simulink model "OpInvDyn"  (Simulink 7.4)
settings: Solver=ode45  StartTime=0.0  StopTime=8  MinStep=0.01  RelTol=1e-3
values from neighbouring files (symbols this model uses):
  Kd = Kp.^0.5*2    [WAMforcecontrol.m]    (also in batchwamobs.m = 50*eye(7); paralelcontrol2R.m = eye(n)*1000)
  Kp = 25*eye(7)    [batchwamobs.m]    (also in paralelcontrol2R.m = eye(n)*2500)
  Md = eye(n)*5    [WAMforcecontrol.m]    (also in feedforward.m = inertia(robot, qd(i,:)); paralelcontrol2R.m = eye(n)*100)
undefined symbols (not defined in the file or in its folder): fdbckOID, p560, splitsignal
libraries: roblocks x2
settings Model: Creator=acolome  LastModifiedBy=acolome

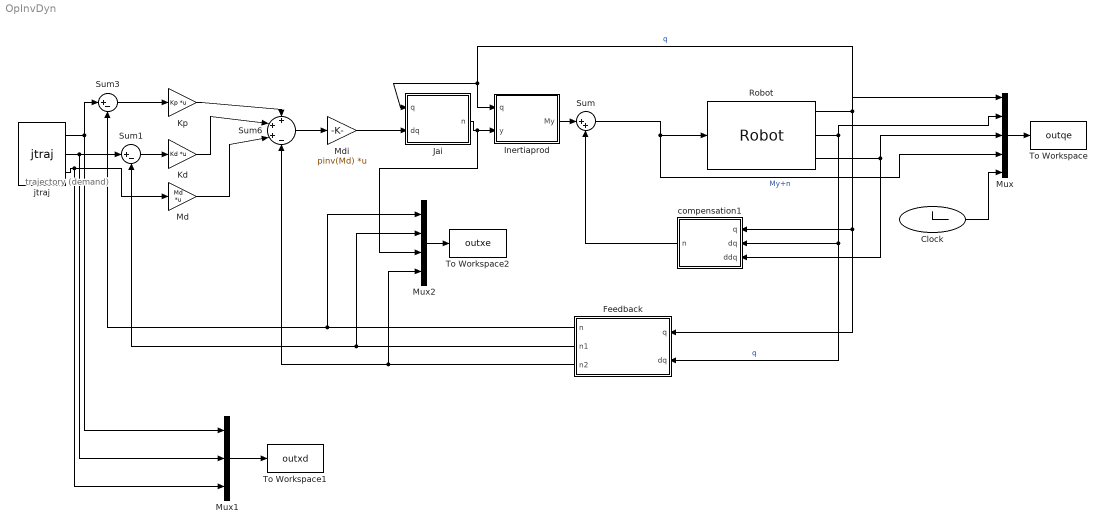
== system OpInvDyn ==
  note: trajectory
      | (demand)
  Clock : Clock
      settings: Decimation=100
  Feedback : Subsystem  mask{robot=p560, g=[0 0 9.81]}
      mask prompts: robot "Robot Object"; g "Gravity"
      mask init:
      | n=robot.n
      mask Display:
      | port_label('output',1,'xe')
      | port_label('output',2,'dxe')
      | port_label('output',3,'dJ(q,dq)·dq')
      | 
      | port_label('input', 1, 'q')
      | port_label('input', 2, 'dq')
  Inertiaprod : Subsystem  mask{robot=p560, g=[0 0 9.81]}
      mask prompts: robot "Robot Object"; g "Gravity"
      mask init:
      | n=robot.n
      mask Display:
      | port_label('output',1,'M(q)y')
      | 
      | port_label('input', 1, 'q')
      | port_label('input', 2, 'y')
  Jai : Subsystem  mask{robot=p560}
      mask prompts: robot "Robot Object"
      mask init:
      | n=robot.n
      mask Display:
      | port_label('output',1,'Jai y')
      | 
      | port_label('input', 1, 'q')
      | port_label('input', 2, 'y')
  Kd : Gain  Gain=Kd  Multiplication=Matrix(K*u)  SaturateOnIntegerOverflow=on  OutDataTypeStr=Inherit: Same as input  ParamDataTypeStr=Inherit: Same as input
  Kp : Gain  Gain=Kp  Multiplication=Matrix(K*u)  SaturateOnIntegerOverflow=on  OutDataTypeStr=Inherit: Same as input  ParamDataTypeStr=Inherit: Same as input
  Md : Gain  Gain=Md  Multiplication=Matrix(K*u)  SaturateOnIntegerOverflow=on  OutDataTypeStr=Inherit: Same as input  ParamDataTypeStr=Inherit: Same as input
  Mdi : Gain  Gain=pinv(Md)  Multiplication=Matrix(K*u)  SaturateOnIntegerOverflow=on  OutDataTypeStr=Inherit: Same as input  ParamDataTypeStr=Inherit: Same as input
  Mux : Mux  Inputs=5
  Mux1 : Mux  Inputs=3
  Mux2 : Mux
  Robot : roblocks/Robot  SystemSampleTime=-1  robot=p560  q0=q0
      link override Integrator1: InitialCondition=q0
  Sum : Sum  Inputs=|++  OutDataType=fixdt(1, 16)  OutScaling=2^0
  Sum1 : Sum  Inputs=|+-  SaturateOnIntegerOverflow=on  InputSameDT=on  OutDataTypeStr=Inherit: Same as first input
  Sum3 : Sum  Inputs=|+-  SaturateOnIntegerOverflow=on  InputSameDT=on  OutDataTypeStr=Inherit: Same as first input
  Sum6 : Sum  Inputs=+++-  OutDataType=fixdt(1, 16)  OutScaling=2^0
  To Workspace : ToWorkspace  VariableName=outqe  SampleTime=-1  SaveFormat=Array
  To Workspace1 : ToWorkspace  VariableName=outxd  SampleTime=-1  SaveFormat=Array
  To Workspace2 : ToWorkspace  VariableName=outxe  SampleTime=-1  SaveFormat=Array
  compensation1 : Subsystem  mask{robot=p560, g=[0 0 9.81]}
      mask prompts: robot "Robot Object"; g "Gravity"
      mask init:
      | n=robot.n
      mask Display:
      | port_label('output',1,'n(q,dq)')
      | 
      | port_label('input', 1, 'q')
      | port_label('input', 2, 'dq')
      | port_label('input', 3, 'ddq')
  jtraj : roblocks/jtraj  SystemSampleTime=-1  q0=x0d  qf=xf  tmax=8
      link override MATLAB Fcn: MATLABFcn=squeeze(interp1(t,q,u))
      link override MATLAB Fcn1: MATLABFcn=squeeze(interp1(t,qd,u))
      link override MATLAB Fcn2: MATLABFcn=squeeze(interp1(t,qdd,u))
  wires:
  Mux/1 -> To Workspace/1
  jtraj/2 -> Sum1/1, Mux1/2
  Sum1/1 -> Kd/1
  Sum3/1 -> Kp/1
  Kd/1 -> Sum6/2
  Kp/1 -> Sum6/1
  Robot/1 -> Mux/1, Feedback/1(q), compensation1/1(q), Inertiaprod/1(q), Jai/1(q)  "q"
  Robot/2 -> Feedback/2(dq), compensation1/2(dq), Mux/2  "q"
  Robot/3 -> Mux/3, compensation1/3(ddq)
  Clock/1 -> Mux/5
  Inertiaprod/1(My) -> Sum/1
  Sum/1 -> Robot/1, Mux/4  "My+n"
  compensation1/1(n) -> Sum/2
  Feedback/1(n) -> Sum3/2, Mux2/1
  jtraj/1 -> Sum3/1, Mux1/1
  Feedback/2(n1) -> Sum1/2, Mux2/2
  Feedback/3(n2) -> Sum6/4, Mux2/4
  Jai/1(n) -> Inertiaprod/2(y), Mux2/3
  jtraj/3 -> Md/1, Mux1/3
  Md/1 -> Sum6/3
  Sum6/1 -> Mdi/1
  Mdi/1 -> Jai/2(dq)
  Mux1/1 -> To Workspace1/1
  Mux2/1 -> To Workspace2/1

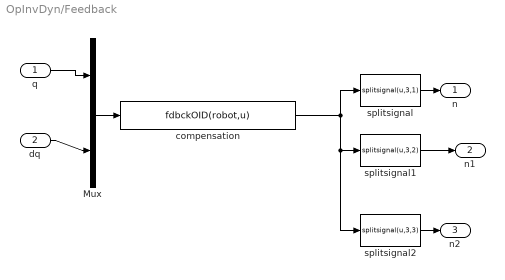
== system OpInvDyn/Feedback ==
  q : Inport  OutDataType=fixdt(1, 16)  OutScaling=2^0
  dq : Inport  Port=2  OutDataType=fixdt(1, 16)  OutScaling=2^0
  Mux : Mux  Inputs=2
  compensation : MATLABFcn  MATLABFcn=fdbckOID(robot,u)  OutputDimensions=3*n
  splitsignal : MATLABFcn  MATLABFcn=splitsignal(u,3,1)  OutputDimensions=n
  splitsignal1 : MATLABFcn  MATLABFcn=splitsignal(u,3,2)  OutputDimensions=n
  splitsignal2 : MATLABFcn  MATLABFcn=splitsignal(u,3,3)  OutputDimensions=n
  n : Outport  OutDataType=fixdt(1, 16)  OutScaling=2^0
  n1 : Outport  Port=2  OutDataType=fixdt(1, 16)  OutScaling=2^0
  n2 : Outport  Port=3  OutDataType=fixdt(1, 16)  OutScaling=2^0
  wires:
  q/1 -> Mux/1
  dq/1 -> Mux/2
  Mux/1 -> compensation/1
  compensation/1 -> splitsignal/1, splitsignal1/1, splitsignal2/1
  splitsignal/1 -> n/1
  splitsignal1/1 -> n1/1
  splitsignal2/1 -> n2/1

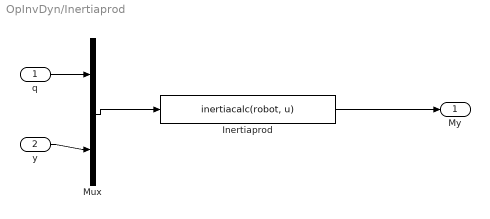
== system OpInvDyn/Inertiaprod ==
  q : Inport  OutDataType=fixdt(1, 16)  OutScaling=2^0
  y : Inport  Port=2  OutDataType=fixdt(1, 16)  OutScaling=2^0
  Inertiaprod : MATLABFcn  MATLABFcn=inertiacalc(robot, u)  OutputDimensions=n
  Mux : Mux  Inputs=2
  My : Outport  OutDataType=fixdt(1, 16)  OutScaling=2^0
  wires:
  Mux/1 -> Inertiaprod/1
  q/1 -> Mux/1
  Inertiaprod/1 -> My/1
  y/1 -> Mux/2

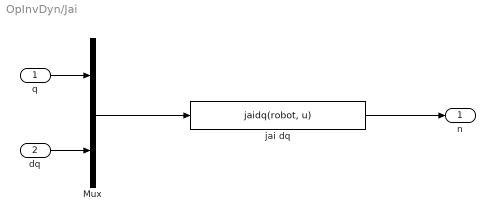
== system OpInvDyn/Jai ==
  q : Inport  OutDataType=fixdt(1, 16)  OutScaling=2^0
  dq : Inport  Port=2  OutDataType=fixdt(1, 16)  OutScaling=2^0
  Mux : Mux  Inputs=2
  jai dq : MATLABFcn  MATLABFcn=jaidq(robot, u)  OutputDimensions=n
  n : Outport  OutDataType=fixdt(1, 16)  OutScaling=2^0
  wires:
  q/1 -> Mux/1
  jai dq/1 -> n/1
  dq/1 -> Mux/2
  Mux/1 -> jai dq/1

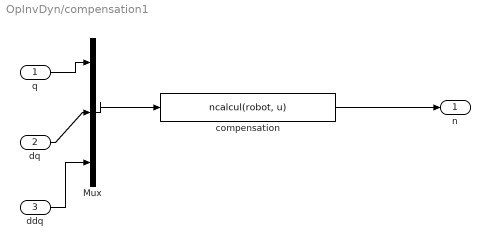
== system OpInvDyn/compensation1 ==
  q : Inport  OutDataType=fixdt(1, 16)  OutScaling=2^0
  dq : Inport  Port=2  OutDataType=fixdt(1, 16)  OutScaling=2^0
  ddq : Inport  Port=3  OutDataType=fixdt(1, 16)  OutScaling=2^0
  Mux : Mux  Inputs=3
  compensation : MATLABFcn  MATLABFcn=ncalcul(robot, u)  OutputDimensions=n
  n : Outport  OutDataType=fixdt(1, 16)  OutScaling=2^0
  wires:
  Mux/1 -> compensation/1
  q/1 -> Mux/1
  compensation/1 -> n/1
  dq/1 -> Mux/2
  ddq/1 -> Mux/3
